simulink model "Copter_Plane_h2g_4_and_1_20210113"  (R2020b)
settings: Solver=ode1  StartTime=0.0  StopTime=50  FixedStep=dt  RelTol=1e-3
values from neighbouring files (symbols this model uses):
  HD = 180/pi    (= 57.2957795131)    [mode_data.m]
undefined symbols (not defined in the file or in its folder): center_WP, GRAVITY_MSS, gyro_x, gyro_y, gyro_z, J, k_aileron, k_aileronL, k_aileronR, k_elevator, k_flap, k_rudder, Kd, Ku, Ld, Ldx, Ldy, Lu, Lux, Luy, m_kg, Newton, pid_vel_xy_derivative, pid_vel_xy_input, pid_vel_xy_integrator, pitch, POSCONTROL_ACC_Z_D, POSCONTROL_ACC_Z_P, POSCONTROL_VEL_XY_D, POSCONTROL_VEL_XY_P, pwm_max, pwm_min, pwm_out, pwm_tail, Qd, QLd, QLdx, QLdy, QLu, QLux, QLuy, Qu, Raphson, roll, tail_tilt, vel_desired, yaw
libraries: shared6dofsys x3, sharedutil x1, simulink x1, aerolibasang x1
(part 1 of 3)
settings Model: xpc_rtwmakecfg_data=_xpcnblib_  PauseTimes=100  Creator=a4327  LastModifiedBy=a4327481
settings DataIOCC: ReturnWorkspaceOutputs=off
settings OptimizationCC: DefaultParameterBehavior=Inlined  UseDivisionForNetSlopeComputation=on  GainParamInheritBuiltInType=on  UseFloatMulNetSlope=on  InlineInvariantSignals=on  PassReuseOutputArgsAs=Individual arguments  ZeroExternalMemoryAtStartup=off  ZeroInternalMemoryAtStartup=off  NoFixptDivByZeroProtection=on  EfficientFloat2IntCast=on  LifeSpan=1  OptimizeBlockOrder=speed  DifferentSizesBufferReuse=on  EfficientTunableParamExpr=on
settings DebuggingCC: ParameterTunabilityLossMsg=error  ArithmeticOperatorsInVariantConditions=warning
settings HardwareCC: ProdBitPerPointer=32  ProdBitPerSizeT=32  ProdBitPerPtrDiffT=32  ProdLargestAtomicFloat=None  ProdWordSize=32  ProdLongLongMode=on  ProdHWDeviceType=Custom Processor->Custom Processor
settings SFSimCC: MATLABDynamicMemAlloc=off  CustomCodeUndefinedFunction=UseInterfaceOnly
settings RTWCC: Description=Embedded Coder  SystemTargetFile=ert.tlc  TemplateMakefile=ert_default_tmf  GenerateReport=on  IncludeHyperlinkInReport=on  LaunchReport=on  GenerateTraceInfo=on  GenerateTraceReport=on  GenerateTraceReportSl=on  GenerateTraceReportSf=on  GenerateTraceReportEml=on  GenerateCodeMetricsReport=on
settings CodeAppCC: ForceParamTrailComments=on  IgnoreCustomStorageClasses=off  OperatorAnnotations=on  SimulinkDataObjDesc=on  SFDataObjDesc=on  CustomSymbolStrGlobalVar=rt$N$M  CustomSymbolStrType=$N$M  CustomSymbolStrFcn=$N$M$F  CustomSymbolStrMacro=$N$M  InsertBlockDesc=on
settings ERTTargetCC: TargetLangStandard=C99 (ISO)  GenerateSampleERTMain=on  IncludeMdlTerminateFcn=off  CombineSignalStateStructs=on  CodeInterfacePackaging=Reusable function  SupportComplex=off  SupportNonInlinedSFcns=on  InlinedParameterPlacement=NonHierarchical  RootIOFormat=Structure reference  ERTCustomFileTemplate=example_file_process.tlc  ERTFilePackagingFormat=CompactWithDataFile

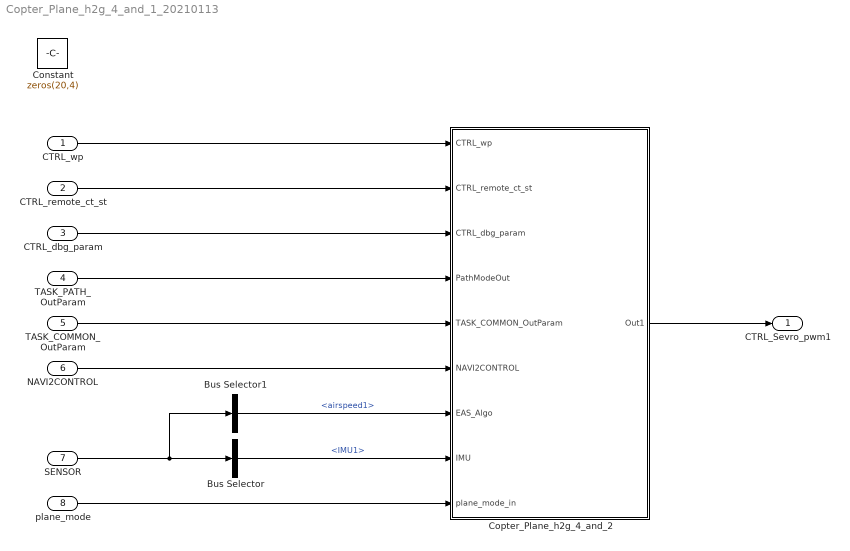
== system Copter_Plane_h2g_4_and_1_20210113 ==
  CTRL_wp : Inport  BusOutputAsStruct=on
  CTRL_remote_ct_st : Inport  Port=2  OutDataTypeStr=Bus: BUS_CTRL_remote_ct_st  BusOutputAsStruct=on
  CTRL_dbg_param : Inport  Port=3  OutDataTypeStr=Bus: BUS_CTRL_dbg_param  BusOutputAsStruct=on
  TASK_PATH_OutParam : Inport  Port=4  OutDataTypeStr=Bus: BUS_TASK_PATH_OutParam  BusOutputAsStruct=on
  TASK_COMMON_OutParam : Inport  Port=5  OutDataTypeStr=Bus: BUS_TASK_COMMON_OutParam  BusOutputAsStruct=on
  NAVI2CONTROL : Inport  Port=6  OutDataTypeStr=Bus: BUS_TO_CONTROL  BusOutputAsStruct=on
  SENSOR : Inport  Port=7  OutDataTypeStr=Bus: BUS_SENSOR
  plane_mode : Inport  Port=8  OutDataTypeStr=Enum: ENUM_plane_mode
  Bus Selector : BusSelector  OutputSignals=IMU1
  Bus Selector1 : BusSelector  OutputSignals=airspeed1
  Constant : Constant  Value=zeros(20,4)
  Copter_Plane_h2g_4_and_2 : Subsystem
  CTRL_Sevro_pwm1 : Outport  OutDataTypeStr=Bus: BUS_CTRL_Sevro_pwm
  wires:
  Copter_Plane_h2g_4_and_2/1(Out1) -> CTRL_Sevro_pwm1/1
  TASK_PATH_OutParam/1 -> Copter_Plane_h2g_4_and_2/4(PathModeOut)
  TASK_COMMON_OutParam/1 -> Copter_Plane_h2g_4_and_2/5(TASK_COMMON_OutParam)
  CTRL_wp/1 -> Copter_Plane_h2g_4_and_2/1(CTRL_wp)
  NAVI2CONTROL/1 -> Copter_Plane_h2g_4_and_2/6(NAVI2CONTROL)
  plane_mode/1 -> Copter_Plane_h2g_4_and_2/9(plane_mode_in)
  SENSOR/1 -> Bus Selector1/1, Bus Selector/1
  CTRL_dbg_param/1 -> Copter_Plane_h2g_4_and_2/3(CTRL_dbg_param)
  CTRL_remote_ct_st/1 -> Copter_Plane_h2g_4_and_2/2(CTRL_remote_ct_st)
  Bus Selector1/1 -> Copter_Plane_h2g_4_and_2/7(EAS_Algo)  "<airspeed1>"
  Bus Selector/1 -> Copter_Plane_h2g_4_and_2/8(IMU)  "<IMU1>"
